simulink model "SeaPort"  (R2023b)
settings: Solver=VariableStepAuto  StartTime=0.0  StopTime=2.0  RelTol=1e-3
(part 3 of 3)

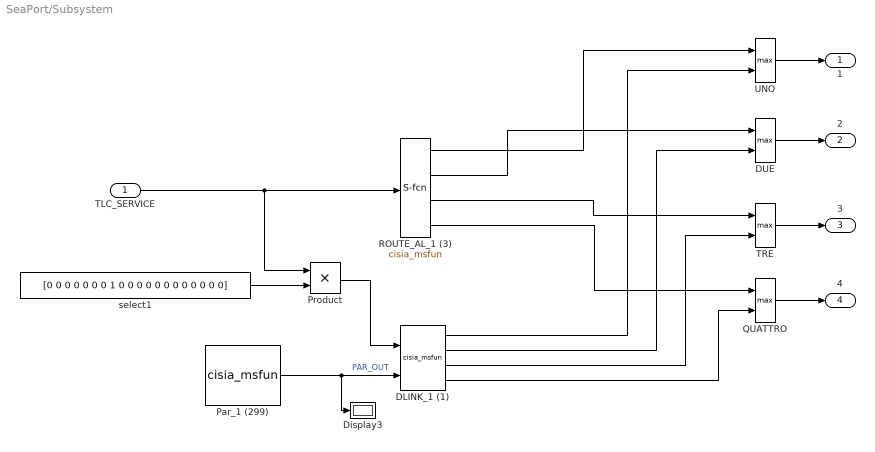
== system SeaPort/Subsystem ==
  TLC_SERVICE : Inport
  DLINK_1 (1) : M-S-Function  FunctionName=cisia_msfun  Parameters=Parameter1, Parameter2, Parameter3, Parameter4, Parameter5, Parameter6, Parameter7  mask(S-function:msfcn_unit_delay){Parameter1='DLINK_1', Parameter2=1, Parameter3='ORO', Parameter4=4, Parameter5=[0 0 0 0 0 0 0 0 0 0 0 0 0 0 0 0 0 0 0 0], Parameter6=20, Parameter7=on}
      mask prompts: Parameter1 "entity name"; Parameter2 "sampling time"; Parameter3 "project"; Parameter4 "number of output links"; Parameter5 "default value for outputs"; Parameter6 "link dimension"; Parameter7 "select link from input"
      mask help: This is a level-2 MATLAB file S-function which demonstrates CISIA entity
      mask Display: disp('DLINK')
  DUE : MinMax  Function=max  Inputs=2
  Display3 : Display
  Par_1 (299) : M-S-Function  FunctionName=cisia_msfun  Parameters=Parameter1, Parameter2, Parameter3, resources, Parameter10, codeupdate, step_received, step_computed, dynamic_computed, step_sended, id_entity, id_project, id_type, name_type, color  mask(S-function:msfcn_unit_delay){Parameter1='Par_1', Parameter2=1, Parameter3='ORO', resources=|, Parameter10=off, codeupdate=off, step_received=, step_computed=, dynamic_computed=, step_sended=PAR_OUT=Route;, id_entity=299, id_project=40, id_type=63, name_type=PARAMETERS, color=#CCCCCC}
      mask resources=|
      | *** INPUT RESOURCES ***
      | NUM_INPUTS 0
      |
      | *** STATE VARIABLES ***
      | NUM_VARIABLES 1
      | Route(NUMERIC)(1)(4)
      |
      | *** OUTPUT RESOURCES ***
      | NUM_OUTPUTS 1
      | PAR_OUT (1)
      mask prompts: Parameter1 "entity name"; Parameter2 "sampling time"; Parameter3 "project"; resources "input resources and state variables"; Parameter10 "Bring state variables to output"; codeupdate "update code from mask"
      mask help: This is a level-2 MATLAB file S-function which demonstrates CISIA entity
      mask DialogControl Container1 Prompt: All parameters
      mask Display: disp('PARAMETERS')
  Product : Product
  QUATTRO : MinMax  Function=max  Inputs=2
  ROUTE_AL_1 (3) : M-S-Function  FunctionName=cisia_msfun  Parameters=Parameter1, Parameter2, Parameter3, Parameter4, Parameter5, Parameter6, Parameter7  mask(S-function:msfcn_unit_delay){Parameter1='ROUTE_AL_1', Parameter2=1, Parameter3='ORO', Parameter4=4, Parameter5=0, Parameter6=20, Parameter7=off}
      mask prompts: Parameter1 "entity name"; Parameter2 "sampling time"; Parameter3 "project"; Parameter4 "number of output links"; Parameter5 "default value for outputs"; Parameter6 "link dimension (unused))"; Parameter7 "select resource elements and output port from input"
      mask help: This is a level-2 MATLAB file S-function which demonstrates CISIA entity
      mask Display: disp('ROUTE')
  TRE : MinMax  Function=max  Inputs=2
  UNO : MinMax  Function=max  Inputs=2
  select1 : Constant  Value=[0 0 0 0 0 0 0 1 0 0 0 0 0 0 0 0 0 0 0 0]
  1 : Outport
  2 : Outport  Port=2
  3 : Outport  Port=3
  4 : Outport  Port=4
  wires:
  TLC_SERVICE/1 -> Product/1, ROUTE_AL_1 (3)/1
  Par_1 (299)/1 -> DLINK_1 (1)/2, Display3/1  "PAR_OUT"
  Product/1 -> DLINK_1 (1)/1
  select1/1 -> Product/2
  UNO/1 -> 1/1
  DUE/1 -> 2/1
  TRE/1 -> 3/1
  QUATTRO/1 -> 4/1
  ROUTE_AL_1 (3)/1 -> UNO/1
  ROUTE_AL_1 (3)/2 -> DUE/1
  ROUTE_AL_1 (3)/3 -> TRE/1
  ROUTE_AL_1 (3)/4 -> QUATTRO/1
  DLINK_1 (1)/1 -> UNO/2
  DLINK_1 (1)/2 -> DUE/2
  DLINK_1 (1)/3 -> TRE/2
  DLINK_1 (1)/4 -> QUATTRO/2

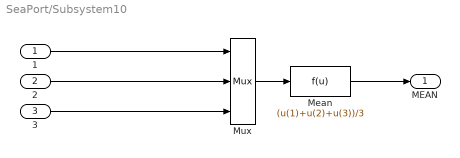
== system SeaPort/Subsystem10 ==
  1 : Inport
  2 : Inport  Port=2
  3 : Inport  Port=3
  Mean : Fcn  Expr=(u(1)+u(2)+u(3))/3
  Mux : Mux  Inputs=3
  MEAN : Outport  VectorParamsAs1DForOutWhenUnconnected=off
  wires:
  1/1 -> Mux/1
  Mux/1 -> Mean/1
  2/1 -> Mux/2
  Mean/1 -> MEAN/1
  3/1 -> Mux/3

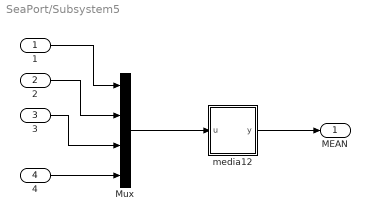
== system SeaPort/Subsystem5 ==
  1 : Inport
  2 : Inport  Port=2
  3 : Inport  Port=3
  4 : Inport  Port=4
  Mux : Mux
  media12 : MATLAB Function  TreatAsAtomicUnit=on
  MEAN : Outport  VectorParamsAs1DForOutWhenUnconnected=off
  wires:
  1/1 -> Mux/1
  Mux/1 -> media12/1(u)
  2/1 -> Mux/2
  media12/1(y) -> MEAN/1
  3/1 -> Mux/3
  4/1 -> Mux/4

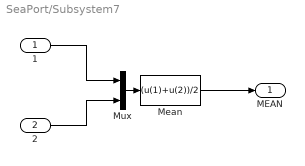
== system SeaPort/Subsystem7 ==
  1 : Inport
  2 : Inport  Port=2
  Mean : Fcn  Expr=(u(1)+u(2))/2
  Mux : Mux  Inputs=2
  MEAN : Outport  VectorParamsAs1DForOutWhenUnconnected=off
  wires:
  1/1 -> Mux/1
  Mux/1 -> Mean/1
  2/1 -> Mux/2
  Mean/1 -> MEAN/1

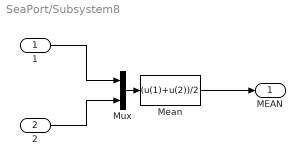
== system SeaPort/Subsystem8 ==
  1 : Inport
  2 : Inport  Port=2
  Mean : Fcn  Expr=(u(1)+u(2))/2
  Mux : Mux  Inputs=2
  MEAN : Outport  VectorParamsAs1DForOutWhenUnconnected=off
  wires:
  1/1 -> Mux/1
  Mux/1 -> Mean/1
  2/1 -> Mux/2
  Mean/1 -> MEAN/1

== matlab function SeaPort/media3 ==
  data: u input; y output
function y = media(u)

y = mean(u);

== matlab function SeaPort/media4 ==
  data: u input; y output
function y = media(u)

y = mean(u);

== matlab function SeaPort/media9 ==
  data: u input; y output
function y = media(u)

y = mean(u);

== matlab function SeaPort/Subsystem5/media12 ==
  data: u input; y output
function y = media(u)

y = mean(u);

== matlab function SeaPort/media2 ==
  data: u input; y output
function y = media(u)

y = mean(u);
